simulink model "IMU_dsPIC_30f4012_AlphaBetaFilter_20Mips_FixedPoints"  (Simulink 6.4)
settings: Solver=FixedStepDiscrete  StartTime=0.0  StopTime=10.0  FixedStep=0.001  RelTol=1e-3
PreLoadFcn:
  | Script_Kalman
values from neighbouring files (symbols this model uses):
  Az = [1 -Ts ;0 1]    [Script_Kalman.m]
  Kz = 1e-3*[.4 ; -.04]    [Script_Kalman.m]
  Ts = .001    (= 0.001)    [Script_Kalman.m]
undefined symbols (not defined in the file or in its folder): DiscIntNeverNeededParam
libraries: simulink x15, dsPICdrivers x10
CloseFcn:
  | rtwprivate ssgencode ModelCloseRequest Autopilote_30f4012
settings Model: Creator=Lubin  LastModifiedBy=Lubin
settings OptimizationCC: InlineParams=on  OptimizeModelRefInitCode=on  LifeSpan=1
settings DebuggingCC: SignalResolutionControl=UseLocalSettings  MultiTaskDSMMsg=error  MultiTaskCondExecSysMsg=warning  MultiTaskRateTransMsg=warning
settings HardwareCC: ProdBitPerInt=16  ProdEndianess=LittleEndian  ProdWordSize=16  ProdHWDeviceType=16-bit Generic
settings RTWCC: SystemTargetFile=dspic.tlc  TemplateMakefile=dspic_pic30_gcc.tmf  PostCodeGenCommand=dsPIC_Compile()  Description=Embedded Target for Microchip dsPIC (real-time)  GenerateReport=on  ProcessScript=dspic_make_rtw_hook  IncludeHyperlinkInReport=on  LaunchReport=on
settings CodeAppCC: IgnoreCustomStorageClasses=off
settings STFCustomTargetCC: TargetFcnLib=ansi_tfl_tmw.mat  GenFloatMathFcnCalls=ANSI_C  ModelReferenceCompliant=off  IncludeMdlTerminateFcn=off  CombineOutputUpdateFcns=on  SuppressErrorStatus=on  ERTCustomFileBanners=on  SupportContinuousTime=off  SupportNonInlinedSFcns=off  SystemTargetFile=dspic.tlc
settings ERTTargetCC: TargetFcnLib=ansi_tfl_tmw.mat  GenFloatMathFcnCalls=ANSI_C  ModelReferenceCompliant=off  CompOptLevelCompliant=off  IncludeMdlTerminateFcn=off  SuppressErrorStatus=on  ModelStepFunctionPrototypeControlCompliant=off  ExtModeMexFile=ext_serial_win32_comm  InlinedParameterPlacement=NonHierarchical  ERTSrcFileBannerTemplate=dsPIC_code_template.cgt  ERTHdrFileBannerTemplate=dsPIC_code_template.cgt  ERTDataSrcFileTemplate=dsPIC_code_template.cgt  ERTDataHdrFileTemplate=dsPIC_code_template.cgt  ERTCustomFileTemplate=dsPIC_main.tlc
settings CustomProperty: DataType=string  Value=C:\PROGRA~1\MATLAB\R2008a\bin\win32\gmake

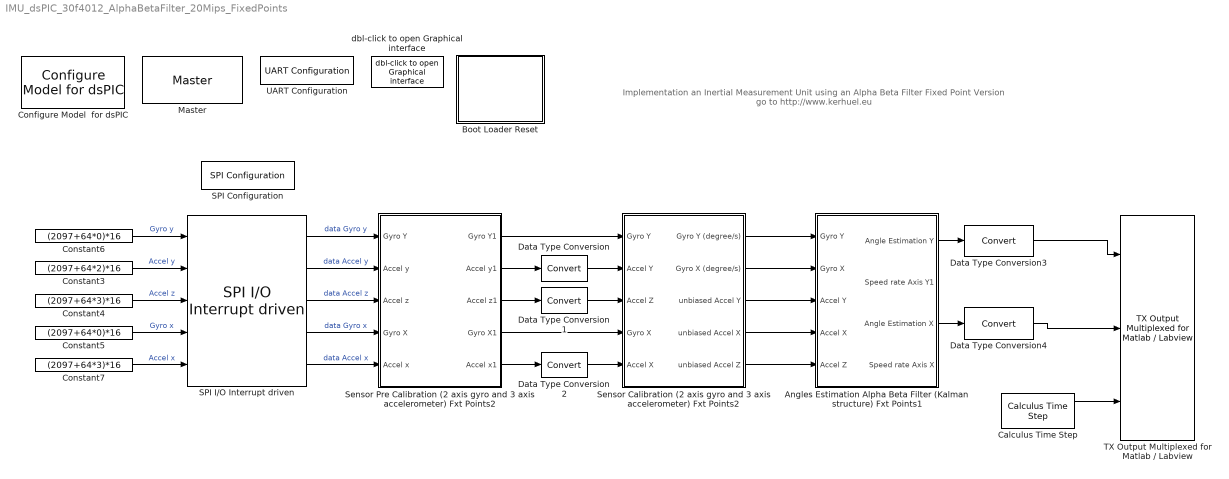
== system IMU_dsPIC_30f4012_AlphaBetaFilter_20Mips_FixedPoints ==
  note: Implementation an Inertial Measurement Unit using an Alpha Beta Filter
      | Fixed Point Version
      | go to http://www.kerhuel.eu
  Angles Estimation Alpha Beta Filter (Kalman structure) Fxt Points1 : Subsystem
  Boot Loader Reset : Subsystem  AncestorBlock=dsPICdrivers/OTHERS/TinyBld Reset
      mask Display: fprintf('TinyBld\nReset')
  Calculus Time Step : dsPICdrivers/OTHERS/Calculus Time Step  Tag=dsPIC_CalculusTimeStep  SampleTime=-1  PR1chk=on
  Configure Model  for dsPIC : dsPICdrivers/Simulink Configuration/Configure Model  for dsPIC
  Constant3 : Constant  Value=(2097+64*2)*16  VectorParams1D=off  OutDataTypeMode=uint16  OutDataType=sfix(16)  OutScaling=2^0  SampleTime=-1
  Constant4 : Constant  Value=(2097+64*3)*16  VectorParams1D=off  OutDataTypeMode=uint16  OutDataType=sfix(16)  OutScaling=2^0  SampleTime=-1
  Constant5 : Constant  Value=(2097+64*0)*16  VectorParams1D=off  OutDataTypeMode=uint16  OutDataType=sfix(16)  OutScaling=2^0  SampleTime=-1
  Constant6 : Constant  Value=(2097+64*0)*16  VectorParams1D=off  OutDataTypeMode=uint16  OutDataType=sfix(16)  OutScaling=2^0  SampleTime=-1
  Constant7 : Constant  Value=(2097+64*3)*16  VectorParams1D=off  OutDataTypeMode=uint16  OutDataType=sfix(16)  OutScaling=2^0  SampleTime=-1
  Data Type Conversion : DataTypeConversion  OutDataTypeMode=int16  OutDataType=sfix(16)  OutScaling=2^0  ConvertRealWorld=Stored Integer (SI)
  Data Type Conversion1 : DataTypeConversion  OutDataTypeMode=int16  OutDataType=sfix(16)  OutScaling=2^0  ConvertRealWorld=Stored Integer (SI)
  Data Type Conversion2 : DataTypeConversion  OutDataTypeMode=int16  OutDataType=sfix(16)  OutScaling=2^0  ConvertRealWorld=Stored Integer (SI)
  Data Type Conversion3 : DataTypeConversion  OutDataTypeMode=int16  OutDataType=sfix(16)  OutScaling=2^0
  Data Type Conversion4 : DataTypeConversion  OutDataTypeMode=int16  OutDataType=sfix(16)  OutScaling=2^0
  Master : dsPICdrivers/Master  Tag=dsPIC_MASTER  Priority=1  TimeStepType=Timer1  picType=30f4012  fcy=20e6  Quartz_33f=5e6  PLLActive_33f=off  fcyDesired_33f=0  tmr1="[1  19999  0]"  tmr1Info="Time Step : 0.001  ;   Error : 0%  PR1=19999"  tmr2345="[0  0  0  0]"  tmr2345cfg=[-1 -1 -1 -1]  IOautoConf=on  typePort="[ 0   0   0   0   0   0   0   0   0   0   0   0   0   0   0   0   0   0   0   0   0   0   0   0   0   0   0   0   0   0   0   0   0   0   0   0   0   0   0   0   0   0   0   0   0   5   4   0   0   0   0   0   0   0   0   0   0   0   0   0   0   0   0   0   0   0   0  21   0  21   0   0  17   0   0   0   0   0   0   0   0   0   0   0   0   0   0   0   0   0   0   0   0   0   0   0   0   0   0   0   0   0   0   0   0   0   0   0   0   0   0   0 ]"  TRIS="[ 65535  65535  65535  65535  65495  65535  65535 ]"  ADPCFG=0  MasterBusyPort=None  MasterOverloadPort=None  FOSC=XT_PLL8  TempProtection_33f=TEMP_ON  FPBOR=PBOR_OFF  PWRT=PWRT_4  MCLR=MCLR_DIS  PowerSave=off
  SPI Configuration : dsPICdrivers/SPI PORT/SPI Configuration  Tag=dsPIC_config_SPI  Priority=2  ConfigurationTime=At boot time (only once)  OrderingInOutPopup=None  SampleTime=-1  Frame_Enable=0  Frame_Sync=0  SPI=1  MODE=MASTER  USER_SCALER=96  StartEnable=Enable  SDO_EN=on  DATA_LENGTH=16 bits  SS_EN=off  SMP=Middle of bit  CKP=high  CKE=Idle to Active  Status="Mode 1  -    Fsck= Not Available"
  SPI I/O Interrupt driven : dsPICdrivers/SPI PORT/SPI I//O Interrupt driven  Tag=dsPIC_SPI_IO_Interrupt  SPI=1  nbrTrame=5  mode=read once - interrupt re-enable after block execution  Disable=on  DATA_LENGTH=16 bits  OrderingInOutPopup=None  SampleTime=.001  T1CSL=E5  T1CSH=None  T2CSL=E5  T2CSH=None  T3CSL=E5  T3CSH=None  T4CSL=E3  T4CSH=None  T5CSL=E3  T5CSH=None  T6CSL=None  T6CSH=None  T7CSL=None  T7CSH=None  T8CSL=None  T8CSH=None  T9CSL=None  T9CSH=None  T10CSL=None  T10CSH=None  T11CSL=None  T11CSH=None  T12CSL=None  T12CSH=None  T13CSL=None  T13CSH=None  T14CSL=None  T14CSH=None  T15CSL=None  T15CSH=None
  Sensor Calibration (2 axis gyro and 3 axis accelerometer) Fxt Points2 : Subsystem
  Sensor Pre Calibration (2 axis gyro and 3 axis accelerometer) Fxt Points2 : Subsystem
  TX Output Multiplexed for Matlab / Labview : dsPICdrivers/Serial PORT/TX Output Multiplexed for Matlab // Labview  Tag=dsPIC_TX_Multiplexed  Priority=5  UART=1  CleverSpreadingChk=on  CleverSpreading=1  CHANNEL=[0 1 2]  CHANNELBLOCKED=[]  CHANNELBLOCKED_BITEWISE=0  Status=OK
  UART Configuration : dsPICdrivers/Serial PORT/UART Configuration  Tag=dsPIC_config_UART  Priority=2  UART=1  proposed_BAUD=115200  ALT_TX_RX=on  InterruptTxWhen=When Transmit Buffer is empty  TXInterruptPri=1  TxBufferSize=32  TXEN=on  InterruptRxWhen=When Receive Buffer is full (contain 4 characters)  RXInterruptPri=1  RxBufferSize=32  BAUD=115200  UxBRG=10  Info="UxBRG = 10   ||  Real Baud : 113636   ||  % error : -1.3573  ||  max 11.3636 Bytes / Step"  RealBaud=0
  dbl-click to open Graphical interface : dsPICdrivers/Serial PORT/dbl-click to open Graphical interface  SystemSampleTime=-1  Nothing=0
  wires:
  Constant6/1 -> SPI I/O Interrupt driven/1  "Gyro y"
  Constant3/1 -> SPI I/O Interrupt driven/2  "Accel y"
  Constant4/1 -> SPI I/O Interrupt driven/3  "Accel z"
  Constant5/1 -> SPI I/O Interrupt driven/4  "Gyro x"
  Constant7/1 -> SPI I/O Interrupt driven/5  "Accel x"
  SPI I/O Interrupt driven/1 -> Sensor Pre Calibration (2 axis gyro and 3 axis accelerometer) Fxt Points2/1(Gyro Y)  "data Gyro y"
  SPI I/O Interrupt driven/2 -> Sensor Pre Calibration (2 axis gyro and 3 axis accelerometer) Fxt Points2/2(Accel y)  "data Accel y"
  SPI I/O Interrupt driven/3 -> Sensor Pre Calibration (2 axis gyro and 3 axis accelerometer) Fxt Points2/3(Accel z)  "data Accel z"
  SPI I/O Interrupt driven/4 -> Sensor Pre Calibration (2 axis gyro and 3 axis accelerometer) Fxt Points2/4(Gyro X)  "data Gyro x"
  SPI I/O Interrupt driven/5 -> Sensor Pre Calibration (2 axis gyro and 3 axis accelerometer) Fxt Points2/5(Accel x)  "data Accel x"
  Angles Estimation Alpha Beta Filter (Kalman structure) Fxt Points1/3(Angle Estimation X) -> Data Type Conversion4/1
  Angles Estimation Alpha Beta Filter (Kalman structure) Fxt Points1/1(Angle Estimation Y) -> Data Type Conversion3/1
  Data Type Conversion/1 -> Sensor Calibration (2 axis gyro and 3 axis accelerometer) Fxt Points2/2(Accel Y)
  Data Type Conversion1/1 -> Sensor Calibration (2 axis gyro and 3 axis accelerometer) Fxt Points2/3(Accel Z)
  Data Type Conversion2/1 -> Sensor Calibration (2 axis gyro and 3 axis accelerometer) Fxt Points2/5(Accel X)
  Sensor Pre Calibration (2 axis gyro and 3 axis accelerometer) Fxt Points2/1(Gyro Y1) -> Sensor Calibration (2 axis gyro and 3 axis accelerometer) Fxt Points2/1(Gyro Y)
  Sensor Pre Calibration (2 axis gyro and 3 axis accelerometer) Fxt Points2/2(Accel y1) -> Data Type Conversion/1
  Sensor Pre Calibration (2 axis gyro and 3 axis accelerometer) Fxt Points2/3(Accel z1) -> Data Type Conversion1/1
  Sensor Pre Calibration (2 axis gyro and 3 axis accelerometer) Fxt Points2/4(Gyro X1) -> Sensor Calibration (2 axis gyro and 3 axis accelerometer) Fxt Points2/4(Gyro X)
  Sensor Pre Calibration (2 axis gyro and 3 axis accelerometer) Fxt Points2/5(Accel x1) -> Data Type Conversion2/1
  Sensor Calibration (2 axis gyro and 3 axis accelerometer) Fxt Points2/2(Gyro X (degree/s)) -> Angles Estimation Alpha Beta Filter (Kalman structure) Fxt Points1/2(Gyro X)
  Sensor Calibration (2 axis gyro and 3 axis accelerometer) Fxt Points2/4(unbiased Accel X) -> Angles Estimation Alpha Beta Filter (Kalman structure) Fxt Points1/4(Accel X)
  Sensor Calibration (2 axis gyro and 3 axis accelerometer) Fxt Points2/5(unbiased Accel Z) -> Angles Estimation Alpha Beta Filter (Kalman structure) Fxt Points1/5(Accel Z)
  Sensor Calibration (2 axis gyro and 3 axis accelerometer) Fxt Points2/3(unbiased Accel Y) -> Angles Estimation Alpha Beta Filter (Kalman structure) Fxt Points1/3(Accel Y)
  Sensor Calibration (2 axis gyro and 3 axis accelerometer) Fxt Points2/1(Gyro Y (degree/s)) -> Angles Estimation Alpha Beta Filter (Kalman structure) Fxt Points1/1(Gyro Y)
  Data Type Conversion3/1 -> TX Output Multiplexed for Matlab / Labview/1
  Data Type Conversion4/1 -> TX Output Multiplexed for Matlab / Labview/2
  Calculus Time Step/1 -> TX Output Multiplexed for Matlab / Labview/3

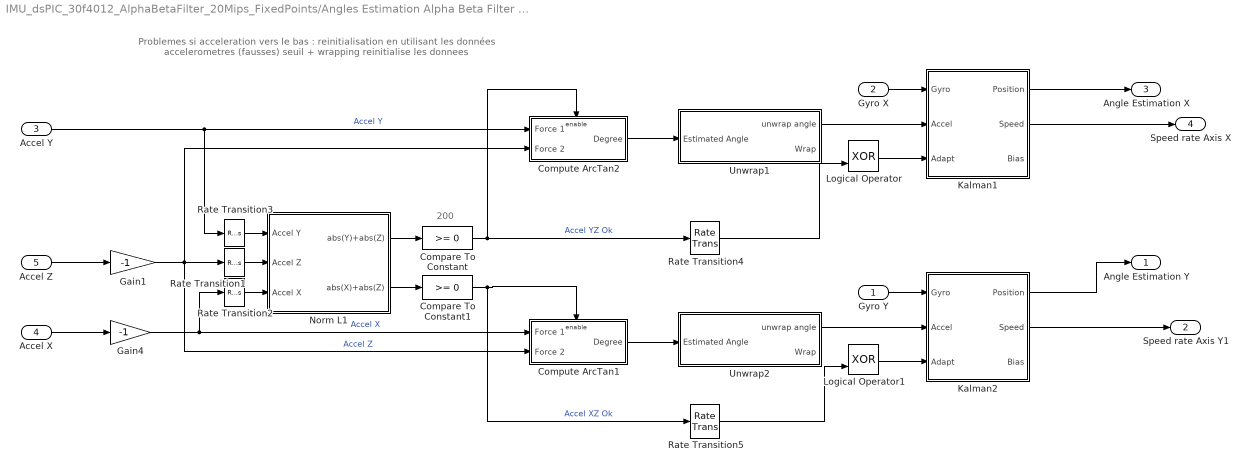
== system IMU_dsPIC_30f4012_AlphaBetaFilter_20Mips_FixedPoints/Angles Estimation Alpha Beta Filter (Kalman structure) Fxt Points1 ==
  note: Problemes si acceleration vers le bas : reinitialisation en utilisant les données accelerometres (fausses)
      | seuil + wrapping reinitialise les donnees
  note: 200
  Gyro Y : Inport
  Gyro X : Inport  Port=2
  Accel Y : Inport  Port=3
  Accel X : Inport  Port=4
  Accel Z : Inport  Port=5
  Compare To Constant : simulink/Logic and Bit Operations/Compare To Constant  SystemSampleTime=-1  relop=>=  const=0  LogicOutDataTypeMode=boolean  ZeroCross=off
  Compare To Constant1 : simulink/Logic and Bit Operations/Compare To Constant  SystemSampleTime=-1  relop=>=  const=0  LogicOutDataTypeMode=boolean  ZeroCross=off
  Compute ArcTan1 : Subsystem
  Compute ArcTan2 : Subsystem
  Gain1 : Gain  Gain=-1  ParameterDataType=sfix(16)  ParameterScaling=2^0  OutDataType=sfix(16)  OutScaling=2^0
  Gain4 : Gain  Gain=-1  ParameterDataType=sfix(16)  ParameterScaling=2^0  OutDataType=sfix(16)  OutScaling=2^0
  Kalman1 : Subsystem
  Kalman2 : Subsystem
  Logical Operator : Logic  Operator=XOR  AllPortsSameDT=off  OutDataTypeMode=boolean
  Logical Operator1 : Logic  Operator=XOR  AllPortsSameDT=off  OutDataTypeMode=boolean
  Norm L1 : Subsystem
  Rate Transition1 : RateTransition  Integrity=off  OutPortSampleTime=.2
  Rate Transition2 : RateTransition  Integrity=off  OutPortSampleTime=.2
  Rate Transition3 : RateTransition  Integrity=off  OutPortSampleTime=.2
  Rate Transition4 : RateTransition  Integrity=off  OutPortSampleTime=.001
  Rate Transition5 : RateTransition  Integrity=off  OutPortSampleTime=.001
  Unwrap1 : Subsystem
  Unwrap2 : Subsystem
  Angle Estimation Y : Outport
  Speed rate Axis Y1 : Outport  Port=2
  Angle Estimation X : Outport  Port=3
  Speed rate Axis X : Outport  Port=4
  wires:
  Gyro Y/1 -> Kalman2/1(Gyro)
  Gyro X/1 -> Kalman1/1(Gyro)
  Accel Y/1 -> Compute ArcTan2/1(Force 1), Rate Transition3/1  "Accel Y"
  Accel X/1 -> Gain4/1
  Compute ArcTan1/1(Degree) -> Unwrap2/1(Estimated Angle)
  Compute ArcTan2/1(Degree) -> Unwrap1/1(Estimated Angle)
  Gain4/1 -> Rate Transition2/1, Compute ArcTan1/1(Force 1)  "Accel X"
  Accel Z/1 -> Gain1/1
  Norm L1/2(abs(X)+abs(Z)) -> Compare To Constant1/1
  Norm L1/1(abs(Y)+abs(Z)) -> Compare To Constant/1
  Compare To Constant/1 -> Rate Transition4/1, Compute ArcTan2/Enable  "Accel YZ Ok"
  Compare To Constant1/1 -> Rate Transition5/1, Compute ArcTan1/Enable  "Accel XZ Ok"
  Kalman1/1(Position) -> Angle Estimation X/1
  Kalman2/1(Position) -> Angle Estimation Y/1
  Rate Transition1/1 -> Norm L1/2(Accel Z)
  Rate Transition2/1 -> Norm L1/3(Accel X)
  Rate Transition3/1 -> Norm L1/1(Accel Y)
  Unwrap1/1(unwrap angle) -> Kalman1/2(Accel)
  Rate Transition4/1 -> Logical Operator/2
  Logical Operator1/1 -> Kalman2/3(Adapt)
  Gain1/1 -> Rate Transition1/1, Compute ArcTan2/2(Force 2), Compute ArcTan1/2(Force 2)  "Accel Z"
  Rate Transition5/1 -> Logical Operator1/2
  Logical Operator/1 -> Kalman1/3(Adapt)
  Unwrap2/1(unwrap angle) -> Kalman2/2(Accel)
  Kalman1/2(Speed) -> Speed rate Axis X/1
  Kalman2/2(Speed) -> Speed rate Axis Y1/1

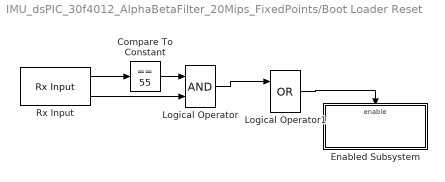
== system IMU_dsPIC_30f4012_AlphaBetaFilter_20Mips_FixedPoints/Boot Loader Reset ==
  Compare To Constant : simulink/Logic and Bit Operations/Compare To Constant  SystemSampleTime=-1  relop===  const=55  LogicOutDataTypeMode=boolean  ZeroCross=off
  Enabled Subsystem : Subsystem  TreatAsAtomicUnit=on
  Logical Operator : Logic  AllPortsSameDT=off  OutDataTypeMode=boolean
  Logical Operator1 : Logic  Operator=OR  AllPortsSameDT=off  OutDataTypeMode=boolean
  Rx Input : dsPICdrivers/Serial PORT/Rx Input  Tag=dsPIC_RX  Priority=5  UART=1  SampleTime=.01  BlockingFctChk=off  OutputDefault=0  IsPresentFlagChk=on
  wires:
  Rx Input/1 -> Compare To Constant/1
  Compare To Constant/1 -> Logical Operator/1
  Rx Input/2 -> Logical Operator/2
  Logical Operator/1 -> Logical Operator1/1
  Logical Operator1/1 -> Enabled Subsystem/Enable

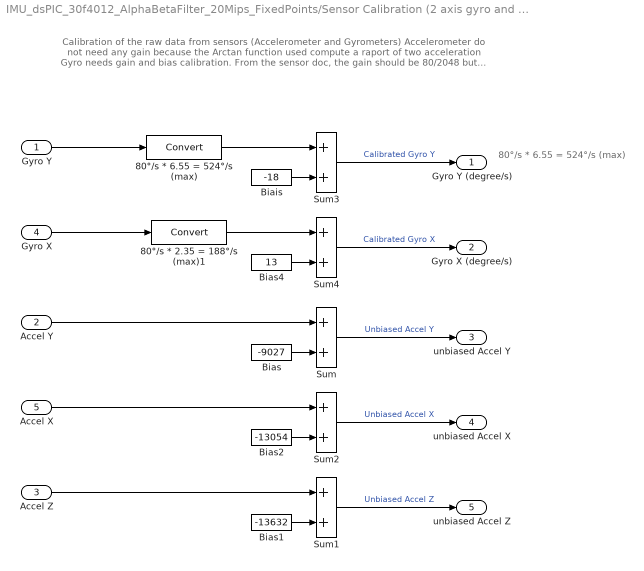
== system IMU_dsPIC_30f4012_AlphaBetaFilter_20Mips_FixedPoints/Sensor Calibration (2 axis gyro and 3 axis accelerometer) Fxt Points2 ==
  note: 80°/s * 6.55 = 524°/s (max)
  note: Calibration of the raw data from sensors (Accelerometer and Gyrometers)
      | Accelerometer do not need any gain because the Arctan function used compute a raport of two acceleration
      | Gyro needs gain and bias calibration. From the sensor doc, the gain should be 80/2048 but...
  Gyro Y : Inport
  Accel Y : Inport  Port=2
  Accel Z : Inport  Port=3
  Gyro X : Inport  Port=4
  Accel X : Inport  Port=5
  80°/s * 2.35 = 188°/s (max)1 : DataTypeConversion  OutDataTypeMode=Specify via dialog  OutDataType=fixdt(1,12,80/2048*2.35,0)  ConvertRealWorld=Stored Integer (SI)
  80°/s * 6.55 = 524°/s (max) : DataTypeConversion  OutDataTypeMode=Specify via dialog  OutDataType=fixdt(1,12,80/2048*6.55,0)  ConvertRealWorld=Stored Integer (SI)
  "Biais " : Constant  Value=-18  OutDataType=sfix(16)  OutScaling=2^0
  Bias : Constant  Value=-9027  OutDataType=sfix(16)  OutScaling=2^0
  Bias1 : Constant  Value=-13632  OutDataType=sfix(16)  OutScaling=2^0
  Bias2 : Constant  Value=-13054  OutDataType=sfix(16)  OutScaling=2^0
  Bias4 : Constant  Value=13  OutDataType=sfix(16)  OutScaling=2^0
  Sum : Sum  OutDataTypeMode=int16  OutDataType=sfix(16)  OutScaling=2^0
  Sum1 : Sum  OutDataTypeMode=int16  OutDataType=sfix(16)  OutScaling=2^0
  Sum2 : Sum  OutDataTypeMode=int16  OutDataType=sfix(16)  OutScaling=2^0
  Sum3 : Sum  OutDataType=sfix(16)  OutScaling=2^0
  Sum4 : Sum  OutDataType=sfix(16)  OutScaling=2^0
  Gyro Y (degree/s) : Outport
  Gyro X (degree/s) : Outport  Port=2
  unbiased Accel Y : Outport  Port=3
  unbiased Accel X : Outport  Port=4
  unbiased Accel Z : Outport  Port=5
  wires:
  Bias/1 -> Sum/2
  Bias1/1 -> Sum1/2
  Bias2/1 -> Sum2/2
  Gyro Y/1 -> 80°/s * 6.55 = 524°/s (max)/1
  Accel Y/1 -> Sum/1
  Sum/1 -> unbiased Accel Y/1  "Unbiased Accel Y"
  Accel Z/1 -> Sum1/1
  Sum1/1 -> unbiased Accel Z/1  "Unbiased Accel Z"
  Gyro X/1 -> 80°/s * 2.35 = 188°/s (max)1/1
  Accel X/1 -> Sum2/1
  Sum2/1 -> unbiased Accel X/1  "Unbiased Accel X"
  80°/s * 6.55 = 524°/s (max)/1 -> Sum3/1
  Sum3/1 -> Gyro Y (degree/s)/1  "Calibrated Gyro Y"
  "Biais "/1 -> Sum3/2
  80°/s * 2.35 = 188°/s (max)1/1 -> Sum4/1
  Sum4/1 -> Gyro X (degree/s)/1  "Calibrated Gyro X"
  Bias4/1 -> Sum4/2

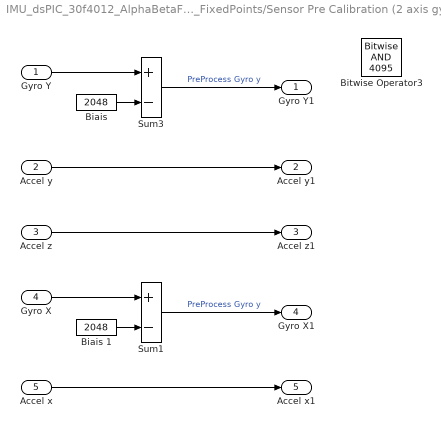
== system IMU_dsPIC_30f4012_AlphaBetaFilter_20Mips_FixedPoints/Sensor Pre Calibration (2 axis gyro and 3 axis accelerometer) Fxt Points2 ==
  Gyro Y : Inport
  Accel y : Inport  Port=2
  Accel z : Inport  Port=3
  Gyro X : Inport  Port=4
  Accel x : Inport  Port=5
  "Biais " : Constant  Value=2048  OutDataType=sfix(16)  OutScaling=2^0
  Biais 1 : Constant  Value=2048  OutDataType=sfix(16)  OutScaling=2^0
  Bitwise Operator3 : simulink/Logic and Bit Operations/Bitwise Operator  logicop=AND  UseBitMask=on  BitMask=4095  BitMaskRealWorld=Stored Integer
  Sum1 : Sum  Inputs=+-  OutDataTypeMode=int16  OutDataType=sfix(16)  OutScaling=2^0
  Sum3 : Sum  Inputs=+-  OutDataTypeMode=int16  OutDataType=sfix(16)  OutScaling=2^0
  Gyro Y1 : Outport
  Accel y1 : Outport  Port=2
  Accel z1 : Outport  Port=3
  Gyro X1 : Outport  Port=4
  Accel x1 : Outport  Port=5
  wires:
  "Biais "/1 -> Sum3/2
  Sum3/1 -> Gyro Y1/1  "PreProcess Gyro y"
  Gyro Y/1 -> Sum3/1
  Accel y/1 -> Accel y1/1
  Accel z/1 -> Accel z1/1
  Biais 1/1 -> Sum1/2
  Sum1/1 -> Gyro X1/1  "PreProcess Gyro y"
  Gyro X/1 -> Sum1/1
  Accel x/1 -> Accel x1/1

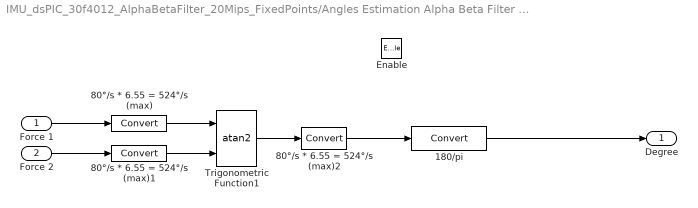
== system IMU_dsPIC_30f4012_AlphaBetaFilter_20Mips_FixedPoints/Angles Estimation Alpha Beta Filter (Kalman structure) Fxt Points1/Compute ArcTan1 ==
  Force 1 : Inport
  Force 2 : Inport  Port=2
  Enable : EnablePort  StatesWhenEnabling=reset
  180/pi : DataTypeConversion  OutDataTypeMode=Specify via dialog  OutDataType=fixdt(1,16,180/pi*2^-12,0)  ConvertRealWorld=Stored Integer (SI)
  80°/s * 6.55 = 524°/s (max) : DataTypeConversion  OutDataTypeMode=single  OutDataType=fixdt(1,12,80/2048*6.55,0)
  80°/s * 6.55 = 524°/s (max)1 : DataTypeConversion  OutDataTypeMode=single  OutDataType=fixdt(1,12,80/2048*6.55,0)
  80°/s * 6.55 = 524°/s (max)2 : DataTypeConversion  OutDataTypeMode=Specify via dialog  OutDataType=fixdt(1,16,12)
  Trigonometric Function1 : Trigonometry  Operator=atan2  OutputSignalType=real
  Degree : Outport
  wires:
  80°/s * 6.55 = 524°/s (max)2/1 -> 180/pi/1
  80°/s * 6.55 = 524°/s (max)1/1 -> Trigonometric Function1/2
  80°/s * 6.55 = 524°/s (max)/1 -> Trigonometric Function1/1
  Force 2/1 -> 80°/s * 6.55 = 524°/s (max)1/1
  Force 1/1 -> 80°/s * 6.55 = 524°/s (max)/1
  180/pi/1 -> Degree/1
  Trigonometric Function1/1 -> 80°/s * 6.55 = 524°/s (max)2/1

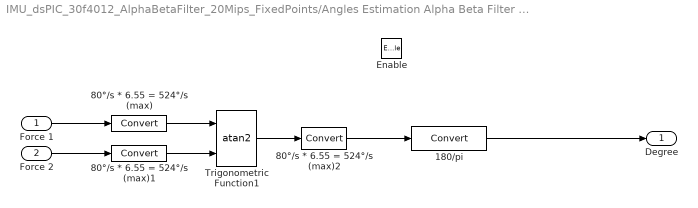
== system IMU_dsPIC_30f4012_AlphaBetaFilter_20Mips_FixedPoints/Angles Estimation Alpha Beta Filter (Kalman structure) Fxt Points1/Compute ArcTan2 ==
  Force 1 : Inport
  Force 2 : Inport  Port=2
  Enable : EnablePort  StatesWhenEnabling=reset
  180/pi : DataTypeConversion  OutDataTypeMode=Specify via dialog  OutDataType=fixdt(1,16,180/pi*2^-12,0)  ConvertRealWorld=Stored Integer (SI)
  80°/s * 6.55 = 524°/s (max) : DataTypeConversion  OutDataTypeMode=single  OutDataType=fixdt(1,12,80/2048*6.55,0)
  80°/s * 6.55 = 524°/s (max)1 : DataTypeConversion  OutDataTypeMode=single  OutDataType=fixdt(1,12,80/2048*6.55,0)
  80°/s * 6.55 = 524°/s (max)2 : DataTypeConversion  OutDataTypeMode=Specify via dialog  OutDataType=fixdt(1,16,12)
  Trigonometric Function1 : Trigonometry  Operator=atan2  OutputSignalType=real
  Degree : Outport
  wires:
  Trigonometric Function1/1 -> 80°/s * 6.55 = 524°/s (max)2/1
  180/pi/1 -> Degree/1
  Force 1/1 -> 80°/s * 6.55 = 524°/s (max)/1
  Force 2/1 -> 80°/s * 6.55 = 524°/s (max)1/1
  80°/s * 6.55 = 524°/s (max)/1 -> Trigonometric Function1/1
  80°/s * 6.55 = 524°/s (max)1/1 -> Trigonometric Function1/2
  80°/s * 6.55 = 524°/s (max)2/1 -> 180/pi/1

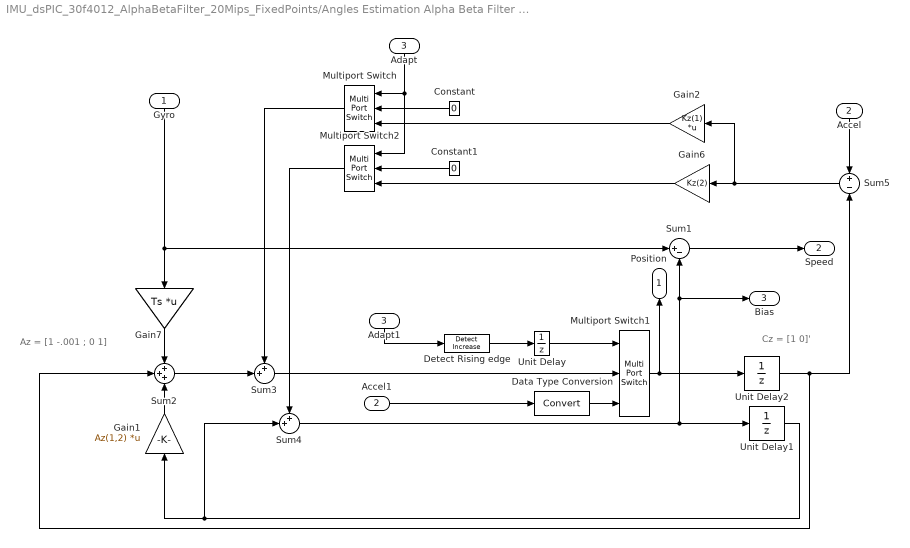
== system IMU_dsPIC_30f4012_AlphaBetaFilter_20Mips_FixedPoints/Angles Estimation Alpha Beta Filter (Kalman structure) Fxt Points1/Kalman1 ==
  note: Cz = [1 0]'
  note: Az = [1 -.001 ; 0 1]
  Gyro : Inport  Orientation=down
  Accel : Inport  Orientation=down  Port=2
  Adapt : Inport  Orientation=down  Port=3
  Accel1 : InportShadow  Port=2  LatchByCopyingInsideSignal=off
  Adapt1 : InportShadow  Orientation=down  Port=3  LatchByCopyingInsideSignal=off
  Constant : Constant  Orientation=left  Value=0  OutDataType=sfix(16)  OutScaling=2^0
  Constant1 : Constant  Orientation=left  Value=0  OutDataType=sfix(16)  OutScaling=2^0
  Data Type Conversion : DataTypeConversion  OutDataType=sfix(16)  OutScaling=2^0
  Detect Rising edge : simulink/Logic and Bit Operations/Detect Increase  SystemSampleTime=-1  vinit=0
  Gain1 : Gain  Orientation=up  Gain=Az(1,2)  Multiplication=Matrix(K*u)  ParameterDataType=sfix(16)  ParameterScaling=2^0  OutDataTypeMode=Specify via dialog  OutDataType=fixdt(1,32,36)
  Gain2 : Gain  Orientation=left  Gain=Kz(1)  Multiplication=Matrix(K*u)  ParameterDataTypeMode=Specify via dialog  ParameterDataType=fixdt(1,32,42)  OutDataTypeMode=Specify via dialog  OutDataType=fixdt(1,16,20)  SaturateOnIntegerOverflow=on
  Gain6 : Gain  Orientation=left  Gain=Kz(2)  ParameterDataTypeMode=Specify via dialog  ParameterDataType=fixdt(1,32,45)  OutDataTypeMode=Specify via dialog  OutDataType=fixdt(1,16,23)  SaturateOnIntegerOverflow=on
  Gain7 : Gain  Orientation=down  Gain=Ts  Multiplication=Matrix(K*u)  ParameterDataType=sfix(16)  ParameterScaling=2^0  OutDataType=sfix(16)  OutScaling=2^0
  Multiport Switch : MultiPortSwitch  Orientation=left  Inputs=2  zeroidx=on
  Multiport Switch1 : MultiPortSwitch  Inputs=2  zeroidx=on
  Multiport Switch2 : MultiPortSwitch  Orientation=left  Inputs=2  zeroidx=on
  Sum1 : Sum  Inputs=|+-  OutDataType=sfix(16)  OutScaling=2^0
  Sum2 : Sum  Inputs=+++  OutDataTypeMode=Specify via dialog  OutDataType=fixdt(1,32,22)
  Sum3 : Sum  Inputs=++|  OutDataTypeMode=Specify via dialog  OutDataType=fixdt(1,32,22)
  Sum4 : Sum  Inputs=++|  OutDataTypeMode=Specify via dialog  OutDataType=fixdt(1,32,26)
  Sum5 : Sum  Orientation=left  Inputs=+-  OutDataTypeMode=Specify via dialog  OutDataType=fixdt(1,16,9)  SaturateOnIntegerOverflow=on
  Unit Delay : UnitDelay  SampleTime=-1
  Unit Delay1 : UnitDelay  SampleTime=-1
  Unit Delay2 : UnitDelay  SampleTime=-1
  Position : Outport  Orientation=up  DataType=Specify via dialog  OutDataType=fixdt(1,32,22)
  Speed : Outport  Port=2  OutDataType=sfix(16)  OutScaling=2^0
  Bias : Outport  Port=3  OutDataType=fixdt(1,32,30)
  wires:
  Adapt1/1 -> Detect Rising edge/1
  Detect Rising edge/1 -> Unit Delay/1
  Constant/1 -> Multiport Switch/2
  Adapt/1 -> Multiport Switch/1, Multiport Switch2/1
  Unit Delay2/1 -> Sum5/2, Sum2/2
  Sum2/1 -> Sum3/2
  Sum5/1 -> Gain6/1, Gain2/1
  Gain7/1 -> Sum2/1
  Accel/1 -> Sum5/1
  Unit Delay/1 -> Multiport Switch1/1
  Sum1/1 -> Speed/1
  Gain1/1 -> Sum2/3
  Gain2/1 -> Multiport Switch/3
  Constant1/1 -> Multiport Switch2/2
  Multiport Switch/1 -> Sum3/1
  Multiport Switch2/1 -> Sum4/1
  Sum3/1 -> Multiport Switch1/2
  Accel1/1 -> Data Type Conversion/1
  Data Type Conversion/1 -> Multiport Switch1/3
  Sum4/1 -> Unit Delay1/1, Sum1/2, Bias/1
  Multiport Switch1/1 -> Unit Delay2/1, Position/1
  Unit Delay1/1 -> Gain1/1, Sum4/2
  Gain6/1 -> Multiport Switch2/3
  Gyro/1 -> Gain7/1, Sum1/1

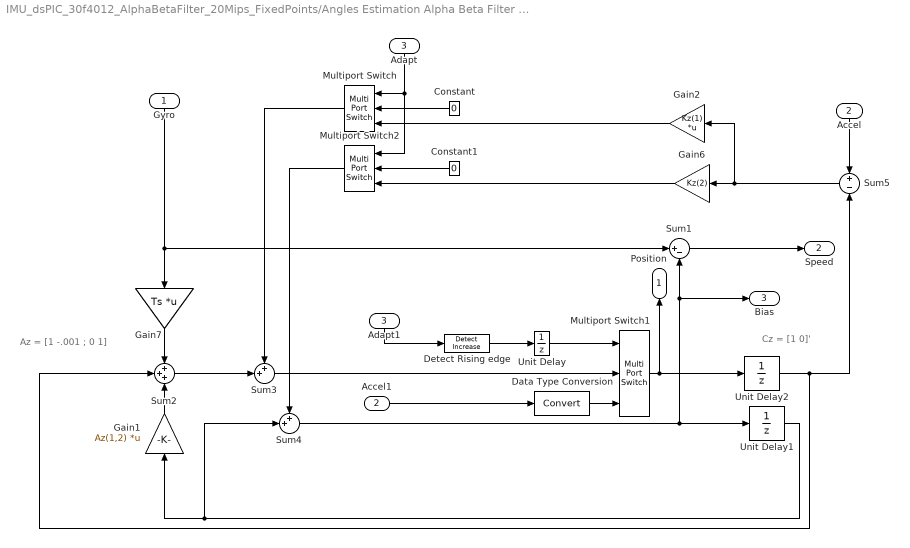
== system IMU_dsPIC_30f4012_AlphaBetaFilter_20Mips_FixedPoints/Angles Estimation Alpha Beta Filter (Kalman structure) Fxt Points1/Kalman2 ==
  note: Az = [1 -.001 ; 0 1]
  note: Cz = [1 0]'
  Gyro : Inport  Orientation=down
  Accel : Inport  Orientation=down  Port=2
  Adapt : Inport  Orientation=down  Port=3
  Accel1 : InportShadow  Port=2  LatchByCopyingInsideSignal=off
  Adapt1 : InportShadow  Orientation=down  Port=3  LatchByCopyingInsideSignal=off
  Constant : Constant  Orientation=left  Value=0  OutDataType=sfix(16)  OutScaling=2^0
  Constant1 : Constant  Orientation=left  Value=0  OutDataType=sfix(16)  OutScaling=2^0
  Data Type Conversion : DataTypeConversion  OutDataType=sfix(16)  OutScaling=2^0
  Detect Rising edge : simulink/Logic and Bit Operations/Detect Increase  SystemSampleTime=-1  vinit=0
  Gain1 : Gain  Orientation=up  Gain=Az(1,2)  Multiplication=Matrix(K*u)  ParameterDataType=sfix(16)  ParameterScaling=2^0  OutDataTypeMode=Specify via dialog  OutDataType=fixdt(1,32,36)
  Gain2 : Gain  Orientation=left  Gain=Kz(1)  Multiplication=Matrix(K*u)  ParameterDataTypeMode=Specify via dialog  ParameterDataType=fixdt(1,32,42)  OutDataTypeMode=Specify via dialog  OutDataType=fixdt(1,16,20)  SaturateOnIntegerOverflow=on
  Gain6 : Gain  Orientation=left  Gain=Kz(2)  ParameterDataTypeMode=Specify via dialog  ParameterDataType=fixdt(1,32,45)  OutDataTypeMode=Specify via dialog  OutDataType=fixdt(1,16,23)  SaturateOnIntegerOverflow=on
  Gain7 : Gain  Orientation=down  Gain=Ts  Multiplication=Matrix(K*u)  ParameterDataType=sfix(16)  ParameterScaling=2^0  OutDataType=sfix(16)  OutScaling=2^0
  Multiport Switch : MultiPortSwitch  Orientation=left  Inputs=2  zeroidx=on
  Multiport Switch1 : MultiPortSwitch  Inputs=2  zeroidx=on
  Multiport Switch2 : MultiPortSwitch  Orientation=left  Inputs=2  zeroidx=on
  Sum1 : Sum  Inputs=|+-  OutDataType=sfix(16)  OutScaling=2^0
  Sum2 : Sum  Inputs=+++  OutDataTypeMode=Specify via dialog  OutDataType=fixdt(1,32,22)
  Sum3 : Sum  Inputs=++|  OutDataTypeMode=Specify via dialog  OutDataType=fixdt(1,32,22)
  Sum4 : Sum  Inputs=++|  OutDataTypeMode=Specify via dialog  OutDataType=fixdt(1,32,26)
  Sum5 : Sum  Orientation=left  Inputs=+-  OutDataTypeMode=Specify via dialog  OutDataType=fixdt(1,16,9)  SaturateOnIntegerOverflow=on
  Unit Delay : UnitDelay  SampleTime=-1
  Unit Delay1 : UnitDelay  SampleTime=-1
  Unit Delay2 : UnitDelay  SampleTime=-1
  Position : Outport  Orientation=up  DataType=Specify via dialog  OutDataType=fixdt(1,32,22)
  Speed : Outport  Port=2  OutDataType=sfix(16)  OutScaling=2^0
  Bias : Outport  Port=3  OutDataType=fixdt(1,32,30)
  wires:
  Gyro/1 -> Sum1/1, Gain7/1
  Gain6/1 -> Multiport Switch2/3
  Unit Delay1/1 -> Sum4/2, Gain1/1
  Multiport Switch1/1 -> Position/1, Unit Delay2/1
  Sum4/1 -> Bias/1, Sum1/2, Unit Delay1/1
  Data Type Conversion/1 -> Multiport Switch1/3
  Accel1/1 -> Data Type Conversion/1
  Sum3/1 -> Multiport Switch1/2
  Multiport Switch2/1 -> Sum4/1
  Multiport Switch/1 -> Sum3/1
  Constant1/1 -> Multiport Switch2/2
  Gain2/1 -> Multiport Switch/3
  Gain1/1 -> Sum2/3
  Sum1/1 -> Speed/1
  Unit Delay/1 -> Multiport Switch1/1
  Accel/1 -> Sum5/1
  Gain7/1 -> Sum2/1
  Sum5/1 -> Gain2/1, Gain6/1
  Sum2/1 -> Sum3/2
  Unit Delay2/1 -> Sum2/2, Sum5/2
  Adapt/1 -> Multiport Switch2/1, Multiport Switch/1
  Constant/1 -> Multiport Switch/2
  Detect Rising edge/1 -> Unit Delay/1
  Adapt1/1 -> Detect Rising edge/1

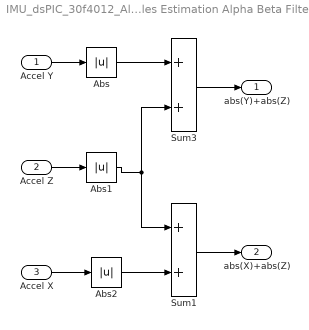
== system IMU_dsPIC_30f4012_AlphaBetaFilter_20Mips_FixedPoints/Angles Estimation Alpha Beta Filter (Kalman structure) Fxt Points1/Norm L1 ==
  Accel Y : Inport
  Accel Z : Inport  Port=2
  Accel X : Inport  Port=3
  Abs : Abs
  Abs1 : Abs
  Abs2 : Abs
  Sum1 : Sum  OutDataType=sfix(16)  OutScaling=2^0
  Sum3 : Sum  OutDataType=sfix(16)  OutScaling=2^0
  abs(Y)+abs(Z) : Outport
  abs(X)+abs(Z) : Outport  Port=2
  wires:
  Abs/1 -> Sum3/1
  Abs1/1 -> Sum1/1, Sum3/2
  Accel Y/1 -> Abs/1
  Accel Z/1 -> Abs1/1
  Sum3/1 -> abs(Y)+abs(Z)/1
  Abs2/1 -> Sum1/2
  Accel X/1 -> Abs2/1
  Sum1/1 -> abs(X)+abs(Z)/1

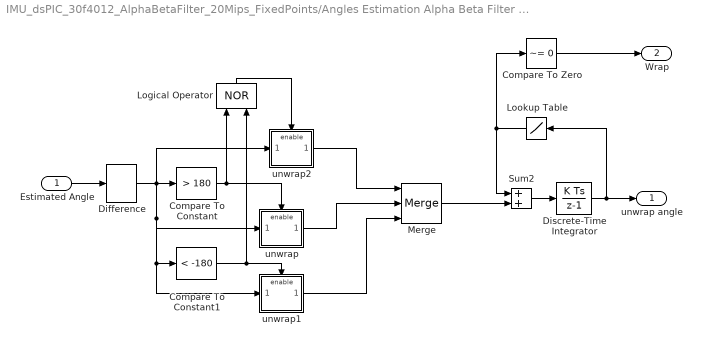
== system IMU_dsPIC_30f4012_AlphaBetaFilter_20Mips_FixedPoints/Angles Estimation Alpha Beta Filter (Kalman structure) Fxt Points1/Unwrap1 ==
  Estimated Angle : Inport
  Compare To Constant : simulink/Logic and Bit Operations/Compare To Constant  SystemSampleTime=-1  relop=>  const=180  LogicOutDataTypeMode=uint8  ZeroCross=off
  Compare To Constant1 : simulink/Logic and Bit Operations/Compare To Constant  SystemSampleTime=-1  relop=<  const=-180  LogicOutDataTypeMode=uint8  ZeroCross=off
  Compare To Zero : simulink/Logic and Bit Operations/Compare To Zero  SystemSampleTime=-1  relop=~=  LogicOutDataTypeMode=uint8  ZeroCross=off
  Difference : simulink/Discrete/Difference  SystemSampleTime=-1  ICPrevInput=0.0  OutDataType=sfix(16)  OutScaling=2^-10  DoSatur=off
  Discrete-Time Integrator : DiscreteIntegrator  gainval=1000  SampleTime=-1  OutDataType=sfix(16)  OutScaling=2^0  ICPrevOutput=DiscIntNeverNeededParam  ICPrevScaledInput=DiscIntNeverNeededParam
  Logical Operator : Logic  Orientation=up  Operator=NOR  AllPortsSameDT=off  OutDataTypeMode=boolean
  Lookup Table : Lookup  Orientation=left  InputValues=[-450 -195 195]  OutputValues=[+360 0 -360]  LookUpMeth=Use Input Below  OutDataType=sfix(16)  OutScaling=2^0
  Merge : Merge  Inputs=3
  Sum2 : Sum  OutDataType=sfix(16)  OutScaling=2^0
  unwrap : Subsystem  TreatAsAtomicUnit=on
  unwrap1 : Subsystem  TreatAsAtomicUnit=on
  unwrap2 : Subsystem  TreatAsAtomicUnit=on
  unwrap angle : Outport
  Wrap : Outport  Port=2
  wires:
  Compare To Zero/1 -> Wrap/1
  Lookup Table/1 -> Compare To Zero/1, Sum2/1
  Merge/1 -> Sum2/2
  Sum2/1 -> Discrete-Time Integrator/1
  Difference/1 -> Compare To Constant/1, unwrap/1(In1), Compare To Constant1/1, unwrap1/1(In1), unwrap2/1(In1)
  Compare To Constant/1 -> Logical Operator/1, unwrap/Enable
  Compare To Constant1/1 -> unwrap1/Enable, Logical Operator/2
  Logical Operator/1 -> unwrap2/Enable
  unwrap2/1(Out1) -> Merge/1
  unwrap/1(Out1) -> Merge/2
  unwrap1/1(Out1) -> Merge/3
  Estimated Angle/1 -> Difference/1
  Discrete-Time Integrator/1 -> Lookup Table/1, unwrap angle/1

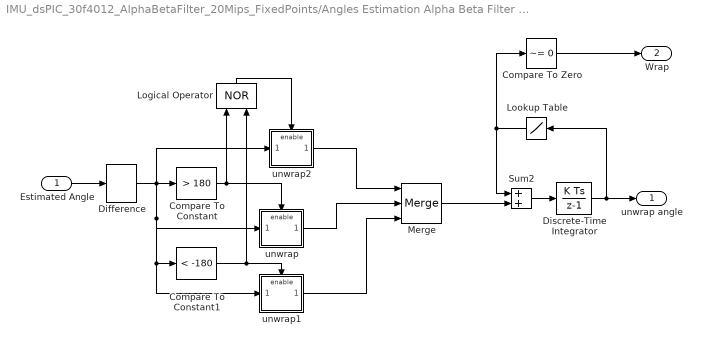
== system IMU_dsPIC_30f4012_AlphaBetaFilter_20Mips_FixedPoints/Angles Estimation Alpha Beta Filter (Kalman structure) Fxt Points1/Unwrap2 ==
  Estimated Angle : Inport
  Compare To Constant : simulink/Logic and Bit Operations/Compare To Constant  SystemSampleTime=-1  relop=>  const=180  LogicOutDataTypeMode=uint8  ZeroCross=off
  Compare To Constant1 : simulink/Logic and Bit Operations/Compare To Constant  SystemSampleTime=-1  relop=<  const=-180  LogicOutDataTypeMode=uint8  ZeroCross=off
  Compare To Zero : simulink/Logic and Bit Operations/Compare To Zero  SystemSampleTime=-1  relop=~=  LogicOutDataTypeMode=uint8  ZeroCross=off
  Difference : simulink/Discrete/Difference  SystemSampleTime=-1  ICPrevInput=0.0  OutDataType=sfix(16)  OutScaling=2^-10  DoSatur=off
  Discrete-Time Integrator : DiscreteIntegrator  gainval=1000  SampleTime=-1  OutDataType=sfix(16)  OutScaling=2^0  ICPrevOutput=DiscIntNeverNeededParam  ICPrevScaledInput=DiscIntNeverNeededParam
  Logical Operator : Logic  Orientation=up  Operator=NOR  AllPortsSameDT=off  OutDataTypeMode=boolean
  Lookup Table : Lookup  Orientation=left  InputValues=[-450 -195 195]  OutputValues=[+360 0 -360]  LookUpMeth=Use Input Below  OutDataType=sfix(16)  OutScaling=2^0
  Merge : Merge  Inputs=3
  Sum2 : Sum  OutDataType=sfix(16)  OutScaling=2^0
  unwrap : Subsystem  TreatAsAtomicUnit=on
  unwrap1 : Subsystem  TreatAsAtomicUnit=on
  unwrap2 : Subsystem  TreatAsAtomicUnit=on
  unwrap angle : Outport
  Wrap : Outport  Port=2
  wires:
  Discrete-Time Integrator/1 -> unwrap angle/1, Lookup Table/1
  Estimated Angle/1 -> Difference/1
  unwrap1/1(Out1) -> Merge/3
  unwrap/1(Out1) -> Merge/2
  unwrap2/1(Out1) -> Merge/1
  Logical Operator/1 -> unwrap2/Enable
  Compare To Constant1/1 -> Logical Operator/2, unwrap1/Enable
  Compare To Constant/1 -> unwrap/Enable, Logical Operator/1
  Difference/1 -> unwrap2/1(In1), unwrap1/1(In1), Compare To Constant1/1, unwrap/1(In1), Compare To Constant/1
  Sum2/1 -> Discrete-Time Integrator/1
  Merge/1 -> Sum2/2
  Lookup Table/1 -> Sum2/1, Compare To Zero/1
  Compare To Zero/1 -> Wrap/1

== system IMU_dsPIC_30f4012_AlphaBetaFilter_20Mips_FixedPoints/Boot Loader Reset/Enabled Subsystem ==
  Enable : EnablePort
  While Iterator Subsystem : Subsystem  TreatAsAtomicUnit=on

== system IMU_dsPIC_30f4012_AlphaBetaFilter_20Mips_FixedPoints/Angles Estimation Alpha Beta Filter (Kalman structure) Fxt Points1/Unwrap1/unwrap ==
  In1 : Inport  OutDataType=sfix(16)  OutScaling=2^0
  Enable : EnablePort
  Bias2 : Constant  Value=-360  OutDataType=sfix(16)  OutScaling=2^0
  Sum2 : Sum  OutDataType=sfix(16)  OutScaling=2^0
  Out1 : Outport  OutDataType=sfix(16)  OutScaling=2^0
  wires:
  In1/1 -> Sum2/1
  Sum2/1 -> Out1/1
  Bias2/1 -> Sum2/2

== system IMU_dsPIC_30f4012_AlphaBetaFilter_20Mips_FixedPoints/Angles Estimation Alpha Beta Filter (Kalman structure) Fxt Points1/Unwrap1/unwrap1 ==
  In1 : Inport  OutDataType=sfix(16)  OutScaling=2^0
  Enable : EnablePort
  Bias2 : Constant  Value=360  OutDataType=sfix(16)  OutScaling=2^0
  Sum2 : Sum  OutDataType=sfix(16)  OutScaling=2^0
  Out1 : Outport  OutDataType=sfix(16)  OutScaling=2^0
  wires:
  In1/1 -> Sum2/1
  Bias2/1 -> Sum2/2
  Sum2/1 -> Out1/1

== system IMU_dsPIC_30f4012_AlphaBetaFilter_20Mips_FixedPoints/Angles Estimation Alpha Beta Filter (Kalman structure) Fxt Points1/Unwrap1/unwrap2 ==
  In1 : Inport  OutDataType=sfix(16)  OutScaling=2^0
  Enable : EnablePort
  Out1 : Outport  OutDataType=sfix(16)  OutScaling=2^0
  wires:
  In1/1 -> Out1/1

== system IMU_dsPIC_30f4012_AlphaBetaFilter_20Mips_FixedPoints/Angles Estimation Alpha Beta Filter (Kalman structure) Fxt Points1/Unwrap2/unwrap ==
  In1 : Inport  OutDataType=sfix(16)  OutScaling=2^0
  Enable : EnablePort
  Bias2 : Constant  Value=-360  OutDataType=sfix(16)  OutScaling=2^0
  Sum2 : Sum  OutDataType=sfix(16)  OutScaling=2^0
  Out1 : Outport  OutDataType=sfix(16)  OutScaling=2^0
  wires:
  Bias2/1 -> Sum2/2
  Sum2/1 -> Out1/1
  In1/1 -> Sum2/1

== system IMU_dsPIC_30f4012_AlphaBetaFilter_20Mips_FixedPoints/Angles Estimation Alpha Beta Filter (Kalman structure) Fxt Points1/Unwrap2/unwrap1 ==
  In1 : Inport  OutDataType=sfix(16)  OutScaling=2^0
  Enable : EnablePort
  Bias2 : Constant  Value=360  OutDataType=sfix(16)  OutScaling=2^0
  Sum2 : Sum  OutDataType=sfix(16)  OutScaling=2^0
  Out1 : Outport  OutDataType=sfix(16)  OutScaling=2^0
  wires:
  Sum2/1 -> Out1/1
  Bias2/1 -> Sum2/2
  In1/1 -> Sum2/1

== system IMU_dsPIC_30f4012_AlphaBetaFilter_20Mips_FixedPoints/Angles Estimation Alpha Beta Filter (Kalman structure) Fxt Points1/Unwrap2/unwrap2 ==
  In1 : Inport  OutDataType=sfix(16)  OutScaling=2^0
  Enable : EnablePort
  Out1 : Outport  OutDataType=sfix(16)  OutScaling=2^0
  wires:
  In1/1 -> Out1/1

== system IMU_dsPIC_30f4012_AlphaBetaFilter_20Mips_FixedPoints/Boot Loader Reset/Enabled Subsystem/While Iterator Subsystem ==
  C1h : simulink/Logic and Bit Operations/Compare To Constant  SystemSampleTime=-1  relop===  const=66  LogicOutDataTypeMode=boolean  ZeroCross=off
  Logical Operator : Logic  Operator=NOT  AllPortsSameDT=off  OutDataTypeMode=boolean
  Rx Input : dsPICdrivers/Serial PORT/Rx Input  Tag=dsPIC_RX  Priority=5  UART=1  SampleTime=-1  BlockingFctChk=on  OutputDefault=0  IsPresentFlagChk=off
  Software RESET : S-Function  Tag=dsPIC_Reset  FunctionName=dsPIC_Reset  EnableBusSupport=off
      mask Description: Reset the microcontroller when input is different from 0
      mask Display:
      | fprintf('Reset');
      | port_label('input', 1 ,'~=0');
  While Iterator : WhileIterator  MaxIters=-1  WhileBlockType=do-while  ResetStates=reset
  wires:
  Logical Operator/1 -> While Iterator/1
  Rx Input/1 -> C1h/1
  C1h/1 -> Software RESET/1, Logical Operator/1
